simulink model "main"  (R2025a)
settings: Solver=VariableStepAuto  StartTime=0.0  StopTime=20  RelTol=1e-3
model workspace (MAT data in the model file):
  AccelNoise = [6.4e-07 6.4e-07 6.4e-07]
  AccelSampleTime = 0.001
  BaroSampleTime = 0.02
  BurnTime = 3.5
  GPSSampleTime = 0.06
  GimbalDelay = 0.02
  GimbalMaxRate = 5
  GimbalMaxSkew = 0.0872665
  Gravity = 9.81
  GyroNoise = [1.1e-08 1.1e-08 1.1e-08]
  GyroSampleTime = 0.001
  IMULocation = [0 0 0]
  InitialCG = [0 0 0]
  Mass = 1
  MaxAttitudeSetpoint = 0.15
  MaxThrust = 25
  MinThrust = 12
  MomentArm = 0.28
  RocketImpulse = 49.6
  RotationMatrix = [1  0  0; 0  1  0; 0  0  1]
  ServoSampleTime = 0.02
  Sig : Simulink.Signal (value not decoded)
  Sig1 : Simulink.Signal (value not decoded)
  VehicleMOI = [0.02  0  0; 0  0.1  0; 0  0  0.1]
  WheelDelay = 0.02
  WheelMOI = 0.0045
  WheelMaxAcceleration = 120
  WheelMaxRate = 500
  WheelSampleTime = 0.05
undefined symbols (not defined in the file): DiscIntNeverNeededParam
libraries: slpidlib x5, aerolibutil x4, aerolibnav x2, aerolibsim3d x2, sensorgpslib x1, sim3dlib x1, matrix_library x1
(part 2 of 2)

== matlab function main/Ignition Control/Apogee Info ==
  settings: updateMethod=DISCRETE  sampleTime=0.01
  data: altitude input; apogeeInfo output; time input
function apogeeInfo = fcn(altitude, time)
    persistent apogee

    apogeeTime = 100000;
    
    if isempty(apogee)
        apogee = 0;
    end

    if altitude > apogee
        apogee = altitude;
    end

    if altitude < apogee - 0.8
        apogeeTime = time;
    end
        
    apogeeInfo = [apogee; apogeeTime];
    return

== matlab function main/State Estimation/Quaternion Integrator ==
  settings: updateMethod=DISCRETE  sampleTime=GyroSampleTime
  data: q_out output; gyroMeasure input size=3; time input size=1
function q_out = quaternion_integrator(gyroMeasure, time)
    persistent last_time
    persistent q_state
    
    if isempty(last_time)
        last_time = 0;
    end
        
    if isempty(q_state)
        q_state = [1, 0, 0, 0];
    end

    dt = time-last_time;
    last_time = time;
        
    quant = quaternion(q_state(1), q_state(2), q_state(3), q_state(4));

    angle = dt * norm(gyroMeasure);
    
    if(norm(gyroMeasure) < 0.0000000000001)
        [w, x, y, z] = parts(normalize(quant));

        q_state = [w, x, y, z];
    
        q_out = [w; x; y; z];
        return;
    end

    axis = gyroMeasure / norm(gyroMeasure);
    r= cos(angle/ double(2));
    i= axis(1) * sin(angle/double(2)) ;
    j= axis(2) * sin(angle/double(2));
    k= axis(3) * sin(angle/double(2));
    dq = quaternion(r,i,j,k);
    new_q = quant * dq;
    [w, x, y, z] = parts(normalize(new_q));
    %fprintf('%.15f\n', parts(new_q));

    q_state = [w, x, y, z];

    q_out = [w; x; y; z];
    return;

== matlab function main/Ignition Control/Ignition Time Calculator ==
  settings: updateMethod=DISCRETE  sampleTime=0.01
  data: apogee input; apogeeTime input; altitude input; ignitionTime output; time input
function ignitionTime = fcn(apogee, apogeeTime, altitude, time)
    persistent ignitionT
    
    if isempty(ignitionT)
        ignitionT = 10;
    end

    if apogeeTime > 999.9
        ignitionTime = 10;
        return
    end

    targetAltitude = apogee * 0.677 - 0.5;

    if altitude < targetAltitude
        if ignitionT > 9.9
            ignitionT = time
        end
    end


        
    ignitionTime = ignitionT;
    return
